simulink model "InductionCookerStateFlow_HarnessIntegrationTest"  (R2023a)
settings: Solver=FixedStepDiscrete  StartTime=0.0  StopTime=60  FixedStep=0.1  RelTol=1e-3  EnableMultiTasking=on
undefined symbols (not defined in the file): D1, P
settings Model: Creator=anton  LastModifiedBy=anton
settings SolverCC: AlgebraicLoopSolver=TrustRegion  AutoInsertRateTranBlk=on
settings DataIOCC: LimitDataPoints=on
settings OptimizationCC: LifeSpan=inf
settings DebuggingCC: UnconnectedInputMsg=warning  UnconnectedOutputMsg=warning  UnconnectedLineMsg=warning  AllowSymbolicDim=off  SFUnexpectedBacktrackingDiag=warning  SFNoUnconditionalDefaultTransitionDiag=warning  SFExecutionAtInitializationDiag=none  ArithmeticOperatorsInVariantConditions=warning
settings ModelReferenceCC: EnableRefExpFcnMdlSchedulingChecks=on
settings SFSimCC: SimUseLocalCustomCode=off  SimGenImportedTypeDefs=on  CustomCodeUndefinedFunction=UseInterfaceOnly
settings RTWCC: RTWUseLocalCustomCode=off  DLArmComputeVersion=19.05
settings CodeAppCC: StateflowObjectComments=on
settings GRTTargetCC: TargetLangStandard=C89/C90 (ANSI)
settings ConfigComp: CovMetricSettings=dw  CovSaveCumulativeToWorkspaceVar=on  CovSaveSingleToWorkspaceVar=on  CovExternalEMLEnable=off  CovSFcnEnable=off

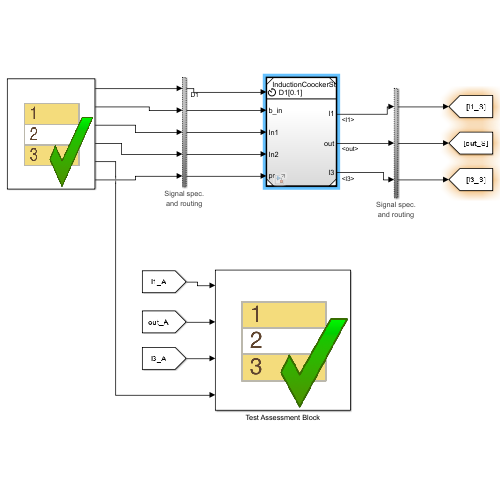
[thumbnail: Simulink's stored preview of the top-level diagram]
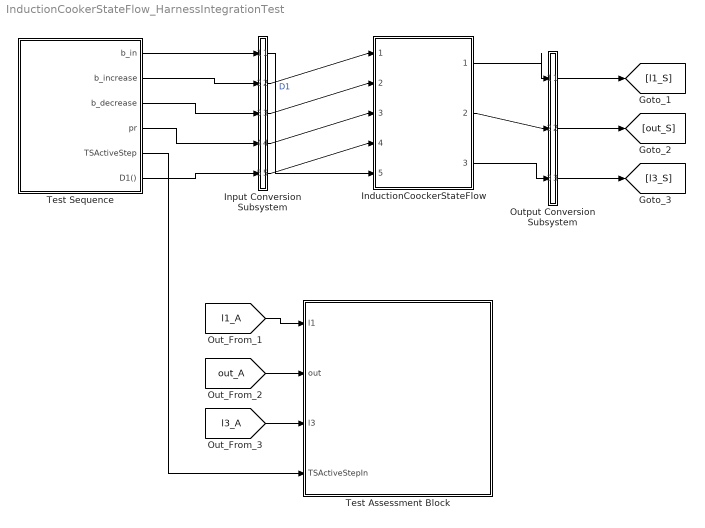
== system InductionCookerStateFlow_HarnessIntegrationTest ==
  InductionCoockerStateFlow : ModelReference  ModelNameDialog=InductionCoockerStateFlow  SimulationMode=Normal  ScheduleRates=on  PortDiscreteRates=[0.1]  CachedPortDiscreteRates=[0.1]  AutoFillPortDiscreteRates=off  ModelEventPortInfo=P:D1[0.1][0][0]  ModelReferenceVersion=1.35
  Input Conversion Subsystem : Subsystem  Tag=__SLT_ICS__  Description=|
      | Signal spec.
      | and routing
      settings: AttributesFormatString=%<Description>
  Output Conversion Subsystem : Subsystem  Tag=__SLT_OCS__  Description=|
      | Signal spec.
      | and routing
      settings: AttributesFormatString=%<Description>
  Test Assessment Block : Test Sequence  Tag=__SLT_ASMT__  TreatAsAtomicUnit=on
  Test Sequence : Test Sequence  TreatAsAtomicUnit=on
  wires:
  [l1_A] -> Test Assessment Block/1(l1)
  [out_A] -> Test Assessment Block/2(out)
  [l3_A] -> Test Assessment Block/3(l3)
  Test Sequence/1(b_in) -> Input Conversion Subsystem/1(Inport_1)
  Test Sequence/2(b_increase) -> Input Conversion Subsystem/2(Inport_2)
  Test Sequence/3(b_decrease) -> Input Conversion Subsystem/3(Inport_3)
  Test Sequence/4(pr) -> Input Conversion Subsystem/4(Inport_4)
  Test Sequence/6(D1()) -> Input Conversion Subsystem/5(Inport_5)
  Output Conversion Subsystem/1(Outport_1) -> [l1_S]
  Output Conversion Subsystem/2(Outport_2) -> [out_S]
  Output Conversion Subsystem/3(Outport_3) -> [l3_S]
  Input Conversion Subsystem/1(Outport_1) -> InductionCoockerStateFlow/5  "D1"
  Input Conversion Subsystem/2(Outport_2) -> InductionCoockerStateFlow/1
  Input Conversion Subsystem/3(Outport_3) -> InductionCoockerStateFlow/2
  Input Conversion Subsystem/4(Outport_4) -> InductionCoockerStateFlow/3
  Input Conversion Subsystem/5(Outport_5) -> InductionCoockerStateFlow/4
  InductionCoockerStateFlow/1 -> Output Conversion Subsystem/1(Inport_1)
  InductionCoockerStateFlow/2 -> Output Conversion Subsystem/2(Inport_2)
  InductionCoockerStateFlow/3 -> Output Conversion Subsystem/3(Inport_3)
  Test Sequence/5(TSActiveStep) -> Test Assessment Block/4(TSActiveStepIn)

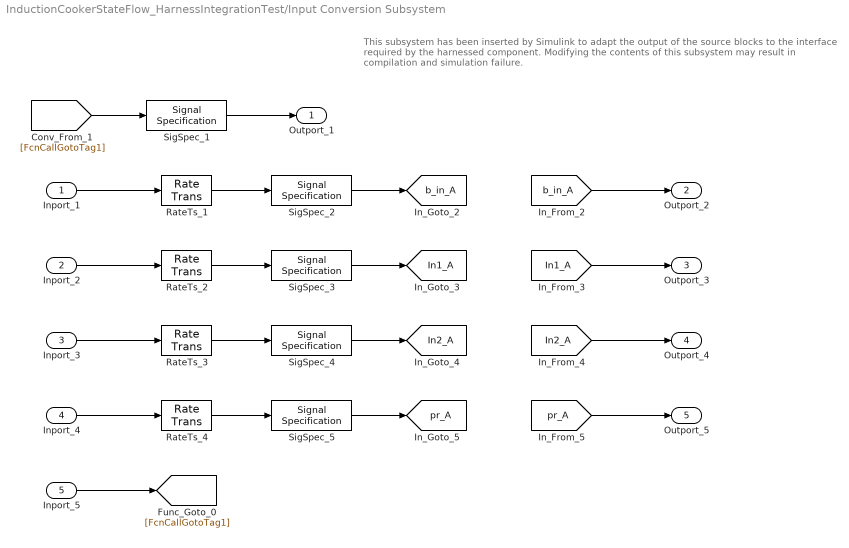
== system InductionCookerStateFlow_HarnessIntegrationTest/Input Conversion Subsystem ==
  note: This subsystem has been inserted by Simulink to adapt the output of the source blocks to the interface required by the harnessed component.
      |  Modifying the contents of this subsystem may result in compilation and simulation failure.
  Inport_1 : Inport
  Inport_2 : Inport  Port=2
  Inport_3 : Inport  Port=3
  Inport_4 : Inport  Port=4
  Inport_5 : Inport  Port=5
  RateTs_{1..4} (4 alike) : RateTransition
  SigSpec_1 : SignalSpecification
  SigSpec_{2..5} (4 alike) : SignalSpecification  OutDataTypeStr=boolean  Dimensions=[1]
  Outport_1 : Outport
  Outport_2 : Outport  Port=2
  Outport_3 : Outport  Port=3
  Outport_4 : Outport  Port=4
  Outport_5 : Outport  Port=5
  tag scope: In1_A=global, In2_A=global, b_in_A=global, pr_A=global
  wires:
  SigSpec_1/1 -> Outport_1/1
  [FcnCallGotoTag1] -> SigSpec_1/1
  [b_in_A] -> Outport_2/1
  SigSpec_2/1 -> [b_in_A]
  RateTs_1/1 -> SigSpec_2/1
  Inport_1/1 -> RateTs_1/1
  [In1_A] -> Outport_3/1
  SigSpec_3/1 -> [In1_A]
  RateTs_2/1 -> SigSpec_3/1
  Inport_2/1 -> RateTs_2/1
  [In2_A] -> Outport_4/1
  SigSpec_4/1 -> [In2_A]
  RateTs_3/1 -> SigSpec_4/1
  Inport_3/1 -> RateTs_3/1
  [pr_A] -> Outport_5/1
  SigSpec_5/1 -> [pr_A]
  RateTs_4/1 -> SigSpec_5/1
  Inport_4/1 -> RateTs_4/1
  Inport_5/1 -> [FcnCallGotoTag1]

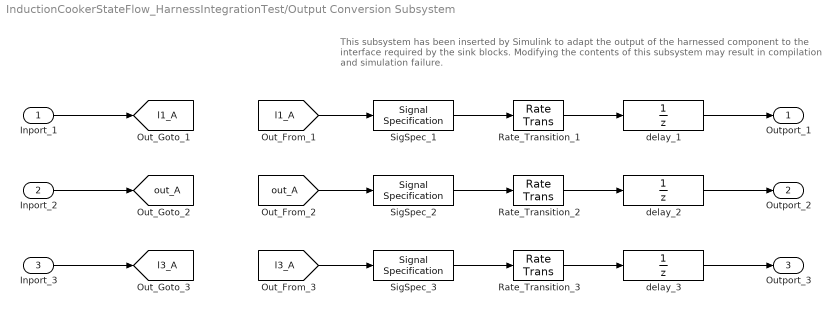
== system InductionCookerStateFlow_HarnessIntegrationTest/Output Conversion Subsystem ==
  note: This subsystem has been inserted by Simulink to adapt the output of the harnessed component to the interface required by the sink blocks.
      |  Modifying the contents of this subsystem may result in compilation and simulation failure.
  Inport_1 : Inport
  Inport_2 : Inport  Port=2
  Inport_3 : Inport  Port=3
  Rate_Transition_1 : RateTransition  OutPortSampleTimeOpt=Inherit
  Rate_Transition_2 : RateTransition  OutPortSampleTimeOpt=Inherit
  Rate_Transition_3 : RateTransition  OutPortSampleTimeOpt=Inherit
  SigSpec_1 : SignalSpecification  OutDataTypeStr=boolean  Dimensions=[1]
  SigSpec_2 : SignalSpecification  OutDataTypeStr=boolean  Dimensions=[1]
  SigSpec_3 : SignalSpecification  OutDataTypeStr=boolean  Dimensions=[1]
  delay_1 : UnitDelay  SampleTime=-1
  delay_2 : UnitDelay  SampleTime=-1
  delay_3 : UnitDelay  SampleTime=-1
  Outport_1 : Outport
  Outport_2 : Outport  Port=2
  Outport_3 : Outport  Port=3
  tag scope: l1_A=global, l3_A=global, out_A=global
  wires:
  Inport_1/1 -> [l1_A]
  [l1_A] -> SigSpec_1/1
  SigSpec_1/1 -> Rate_Transition_1/1
  Rate_Transition_1/1 -> delay_1/1
  delay_1/1 -> Outport_1/1
  Inport_2/1 -> [out_A]
  [out_A] -> SigSpec_2/1
  SigSpec_2/1 -> Rate_Transition_2/1
  Rate_Transition_2/1 -> delay_2/1
  delay_2/1 -> Outport_2/1
  Inport_3/1 -> [l3_A]
  [l3_A] -> SigSpec_3/1
  SigSpec_3/1 -> Rate_Transition_3/1
  Rate_Transition_3/1 -> delay_3/1
  delay_3/1 -> Outport_3/1

== stateflow chart InductionCookerStateFlow_HarnessIntegrationTest/Test Assessment Block ==
  state Scenario_1
    state Run
      state VerifyInit
        verify(~l1 & ~out & ~l3)
      state VerifyStep1
        verify(l1 & ~out & ~l3)
      state VerifyStep2
        verify(l1 & ~out & ~l3)
      state VerifyStep3
        verify(l1 & ~out & ~l3)
      state VerifyStep4
        verify(l1 & ~out & ~l3)
      state VerifyStep5
        state VerifyStep5_1
          verify(l1 & ~out & ~l3)
        state VerifyStep5_2
          verify(l1 & out & ~l3)
        state VerifyStep5_3
          verify(l1 & ~out & ~l3)
        (default) -> VerifyStep5_1
        VerifyStep5_1 -> VerifyStep5_2 : [
            | after(4.8, sec)
            | ]
        VerifyStep5_2 -> VerifyStep5_3 : [
            | after(2, sec)
            | ]
        VerifyStep5_3 -> VerifyStep5_2 : [
            | after(2, sec)
            | ]
      state VerifyStep6
        verify(l1 & out & ~l3)
      state VerifyStep7
        state VerifyStep7_1
          verify(l1 & out & ~l3)
        state VerifyStep7_2
          verify(l1 & ~out & ~l3)
        (default) -> VerifyStep7_1
        VerifyStep7_1 -> VerifyStep7_2 : [
            | after(0.8, sec)
            | ]
      state VerifyStep8
        state VerifyStep8_1
          verify(l1 & ~out & l3)
        state VerifyStep8_3
          verify(l1 & out & l3)
        state VerifyStep8_4
          verify(l1 & ~out & l3)
        state VerifyStep8_5
          verify(l1 & out & l3)
        (default) -> VerifyStep8_1
        VerifyStep8_1 -> VerifyStep8_3 : [
            | after(1, sec)
            | ]
        VerifyStep8_3 -> VerifyStep8_4 : [
            | after(2, sec)
            | ]
        VerifyStep8_4 -> VerifyStep8_5 : [
            | after(2, sec)
            | ]
      state VerifyStep9
        state VerifyStep9_1
          verify(l1 & ~out & ~l3)
        state VerifyStep9_2
          verify(l1 & out & ~l3)
        (default) -> VerifyStep9_1
        VerifyStep9_1 -> VerifyStep9_2 : [
            | after(1, sec)
            | ]
        VerifyStep9_2 -> VerifyStep9_1 : [
            | after(1, sec)
            | ]
      state VerifyStep10
        state VerifyStep10_1
          verify(l1 & ~out & l3)
        state VerifyStep10_2
          verify(l1 & out & l3)
        (default) -> VerifyStep10_1
        VerifyStep10_1 -> VerifyStep10_2 : [
            | after(1, sec)
            | ]
        VerifyStep10_2 -> VerifyStep10_1 : [
            | after(1, sec)
            | ]
      state VerifyStep11
        verify(l1 & ~out & ~l3)
      state VerifyStep12
        state VerifyStep12_1
          verify(l1 & ~out & ~l3)
        state VerifyStep12_3
          verify(~l1 & ~out & ~l3)
        (default) -> VerifyStep12_1
        VerifyStep12_1 -> VerifyStep12_3 : [
            | after(1, sec)
            | ]
      state VerifyStep13
        verify(~l1 & ~out & ~l3)
      state step_1_2
      Run -> (junction 271)
      (default) -> (junction 271)
      (junction 271) -> (junction 272) [order 1] : [TSActiveStepIn == TSActiveStepEnumHarnessIntegrationTest.Init
          | ]
      (junction 272) -> VerifyInit [order 1] : [~in(Scenario_1.Run.VerifyInit)]
      (junction 271) -> (junction 280) [order 2]
      (junction 272) -> (junction 275) [order 2]
      (junction 280) -> (junction 281) [order 1] : [TSActiveStepIn == TSActiveStepEnumHarnessIntegrationTest.Step1
          | ]
      (junction 281) -> VerifyStep1 [order 1] : [~in(Scenario_1.Run.VerifyStep1)]
      (junction 280) -> (junction 288) [order 2]
      (junction 281) -> (junction 284) [order 2]
      (junction 288) -> (junction 289) [order 1] : [TSActiveStepIn == TSActiveStepEnumHarnessIntegrationTest.Step2
          | ]
      (junction 289) -> VerifyStep2 [order 1] : [~in(Scenario_1.Run.VerifyStep2)]
      (junction 288) -> (junction 296) [order 2]
      (junction 289) -> (junction 292) [order 2]
      (junction 296) -> (junction 297) [order 1] : [TSActiveStepIn == TSActiveStepEnumHarnessIntegrationTest.Step3
          | ]
      (junction 297) -> VerifyStep3 [order 1] : [~in(Scenario_1.Run.VerifyStep3)]
      (junction 296) -> (junction 304) [order 2]
      (junction 297) -> (junction 300) [order 2]
      (junction 304) -> (junction 305) [order 1] : [TSActiveStepIn == TSActiveStepEnumHarnessIntegrationTest.Step4
          | ]
      (junction 305) -> VerifyStep4 [order 1] : [~in(Scenario_1.Run.VerifyStep4)]
      (junction 304) -> (junction 312) [order 2]
      (junction 305) -> (junction 308) [order 2]
      (junction 312) -> (junction 313) [order 1] : [TSActiveStepIn == TSActiveStepEnumHarnessIntegrationTest.Step5
          | ]
      (junction 313) -> VerifyStep5 [order 1] : [~in(Scenario_1.Run.VerifyStep5)]
      (junction 312) -> (junction 327) [order 2]
      (junction 313) -> (junction 316) [order 2]
      (junction 327) -> (junction 328) [order 1] : [TSActiveStepIn == TSActiveStepEnumHarnessIntegrationTest.Step6
          | ]
      (junction 328) -> VerifyStep6 [order 1] : [~in(Scenario_1.Run.VerifyStep6)]
      (junction 327) -> (junction 335) [order 2]
      (junction 328) -> (junction 331) [order 2]
      (junction 335) -> (junction 336) [order 1] : [TSActiveStepIn == TSActiveStepEnumHarnessIntegrationTest.Step7
          | ]
      (junction 336) -> VerifyStep7 [order 1] : [~in(Scenario_1.Run.VerifyStep7)]
      (junction 335) -> (junction 349) [order 2]
      (junction 336) -> (junction 339) [order 2]
      (junction 349) -> (junction 350) [order 1] : [TSActiveStepIn == TSActiveStepEnumHarnessIntegrationTest.Step8
          | ]
      (junction 350) -> VerifyStep8 [order 1] : [~in(Scenario_1.Run.VerifyStep8)]
      (junction 349) -> (junction 365) [order 2]
      (junction 350) -> (junction 353) [order 2]
      (junction 365) -> (junction 366) [order 1] : [TSActiveStepIn == TSActiveStepEnumHarnessIntegrationTest.Step9
          | ]
      (junction 366) -> VerifyStep9 [order 1] : [~in(Scenario_1.Run.VerifyStep9)]
      (junction 365) -> (junction 379) [order 2]
      (junction 366) -> (junction 369) [order 2]
      (junction 379) -> (junction 380) [order 1] : [TSActiveStepIn == TSActiveStepEnumHarnessIntegrationTest.Step10
          | ]
      (junction 380) -> VerifyStep10 [order 1] : [~in(Scenario_1.Run.VerifyStep10)]
      (junction 379) -> (junction 393) [order 2]
      (junction 380) -> (junction 383) [order 2]
      (junction 393) -> (junction 394) [order 1] : [TSActiveStepIn == TSActiveStepEnumHarnessIntegrationTest.Step11
          | ]
      (junction 394) -> VerifyStep11 [order 1] : [~in(Scenario_1.Run.VerifyStep11)]
      (junction 393) -> (junction 401) [order 2]
      (junction 394) -> (junction 397) [order 2]
      (junction 401) -> (junction 402) [order 1] : [TSActiveStepIn == TSActiveStepEnumHarnessIntegrationTest.Step12
          | ]
      (junction 402) -> VerifyStep12 [order 1] : [~in(Scenario_1.Run.VerifyStep12)]
      (junction 401) -> (junction 415) [order 2]
      (junction 402) -> (junction 405) [order 2]
      (junction 415) -> (junction 416) [order 1] : [TSActiveStepIn == TSActiveStepEnumHarnessIntegrationTest.Step13
          | ]
      (junction 416) -> VerifyStep13 [order 1] : [~in(Scenario_1.Run.VerifyStep13)]
      (junction 416) -> (junction 419) [order 2]
      (junction 423) -> (junction 424)
      (junction 424) -> step_1_2 [order 1] : [~in(Scenario_1.Run.step_1_2)]
      (junction 424) -> (junction 427) [order 2]
      (junction 415) -> (junction 423) [order 2]
    (default) -> Run
  (default) -> Scenario_1 : {assert(Active_Scenario_Index == 1,'The value of Scenario Parameter ''Active_Scenario_Index'' is not valid. Use the index of the scenario to specify it.')}
  data: l1 input boolean size=[1]; out input boolean size=[1]; l3 input boolean size=[1]; TSActiveStepIn input; Active_Scenario_Index parameter =1

== stateflow chart InductionCookerStateFlow_HarnessIntegrationTest/Test Sequence ==
  settings: updateMethod=DISCRETE  sampleTime=0.1
  state Scenario_1
    state Init
      %% Initialize data outputs.
      b_in = true;
      b_increase= true;
      b_decrease= true;
      pr = true;
      send(D1);
      settings: description=|
          | Condizione iniziale in cui il dispositivo
          | è spento: tutti i pulsanti non sono
          | premuti e la pentola non è presente.
    state Step1
      b_in = false;
      b_increase= true;
      b_decrease= true;
      pr = true;
      send(D1);
      settings: description=|
          | Condizione in cui il pulsante di
          | accensione viene premuto per la messa
          | in funzione del sistema.
    state Step2
      b_in = true;
      b_increase= true;
      b_decrease= true;
      pr = true;
      send(D1);
      settings: description=|
          | Condizione in cui il pulsante di
          | accensione viene rilasciato.
    state Step3
      b_in = true;
      b_increase= true;
      b_decrease= true;
      pr = false;
      send(D1);
      settings: description=|
          | Condizione in cui viene posizionata
          | la pentola.
    state Step4
      b_in = true;
      b_increase= false;
      b_decrease= true;
      pr = false;
      send(D1);
      settings: description=|
          | Condizione in cui viene premuto il
          | pulsante per l'aumento della potenza
          | per almeno 1 secondo.
    state Step5
      b_in = true;
      b_increase= true;
      b_decrease= true;
      pr = false;
      send(D1);
      settings: description=|
          | Condizione in cui il pulsante per
          | l'aumento della potenza viene rilasciato
          | e si attendono i 5 secondi necessari
          | affinché il fornello inizia ad erogare
          | 300W di potenza e il led associato
          | lampeggia con periodo di 2000ms.
    state Step6
      b_in = true;
      b_increase= false;
      b_decrease= true;
      pr = false;
      send(D1);
      settings: description=|
          | Condizione in cui viene premuto il
          | pulsante per l'aumento della potenza
          | per almeno 1 secondo.
    state Step7
      b_in = true;
      b_increase= true;
      b_decrease= true;
      pr = false;
      send(D1);
      settings: description=|
          | Condizione in cui il pulsante per
          | l'aumento della potenza viene rilasciato.
    state Step8
      b_in = true;
      b_increase= true;
      b_decrease= true;
      pr = true;
      send(D1);
      settings: description=|
          | Condizione in cui la pentola viene
          | rimossa prima dello scdere dei 5
          | secondi per il cambio della potenza.
    state Step9
      b_in = true;
      b_increase= true;
      b_decrease= true;
      pr = false;
      send(D1);
      settings: description=|
          | Condizione in cui la pentola viene
          | riposizionata entro i 10 secondi
          | di anomalia e si ha l'effettivo cambio
          | di potenza a 500W.
    state Step10
      b_in = true;
      b_increase= true;
      b_decrease= true;
      pr = true;
      send(D1);
      settings: description=|
          | Condizione in cui la pentola viene rimossa
          | definitivamente per la durata dell'intera
          | anomalia.
    state Step11
      b_in = true;
      b_increase= true;
      b_decrease= true;
      pr = true;
      send(D1);
      settings: description=|
          | Condizione in cui la pentola non è
          | presente e tutti i pulsanti non sono
          | premuti. In particolare, il fornello è
          | acceso alla potenza di 0W, ovvero è
          | inattivo.
    state Step12
      b_in = false;
      b_increase= true;
      b_decrease= true;
      pr = true;
      send(D1);
      settings: description=|
          | Condizione in cui il pulsante di spegimento
          | viene premuto per almeno 1 secondo.
    state Step13
      b_in = true;
      b_increase= true;
      b_decrease= true;
      pr = true;
      send(D1);
      settings: description=|
          | Condizione in cui il dipositivo è
          | completamente spento, riconducendoci
          | così alla situazione di partenza.
    (default) -> Init
    Init -> Step1 : [
        | true
        | ]
    Step1 -> Step2 : [
        | true
        | ]
    Step2 -> Step3 : [
        | after(3, sec)
        | ]
    Step3 -> Step4 : [
        | after(2, sec)
        | ]
    Step4 -> Step5 : [
        | after(1.2, sec)
        | ]
    Step5 -> Step6 : [
        | after(12.8, sec)
        | ]
    Step6 -> Step7 : [
        | after(1.2, sec)
        | ]
    Step7 -> Step8 : [
        | after(1.8, sec)
        | ]
    Step8 -> Step9 : [
        | after(6, sec)
        | ]
    Step9 -> Step10 : [
        | after(6, sec)
        | ]
    Step10 -> Step11 : [
        | after(10, sec)
        | ]
    Step11 -> Step12 : [
        | after(5, sec)
        | ]
    Step12 -> Step13 : [
        | after(1.2, sec)
        | ]
  (default) -> Scenario_1 : {assert(Active_Scenario_Index == 1,'The value of Scenario Parameter ''Active_Scenario_Index'' is not valid. Use the index of the scenario to specify it.')}
  data: b_in output boolean size=[1]; b_increase output boolean size=[1]; b_decrease output boolean size=[1]; pr output boolean size=[1]; TSActiveStep output Enum: TSActiveStepEnumHarnessIntegrationTest; Active_Scenario_Index parameter =1
  events: D1 output FUNCTION_CALL_EVENT
